simulink library "AvgModels.r2022"  (R2021b)
settings: Solver=ode45  StartTime=0.0  StopTime=10.0  RelTol=1e-3  EnableMultiTasking=on
libraries: simulink x8, $bdroot x8, slpidlib x3
(part 2 of 2)

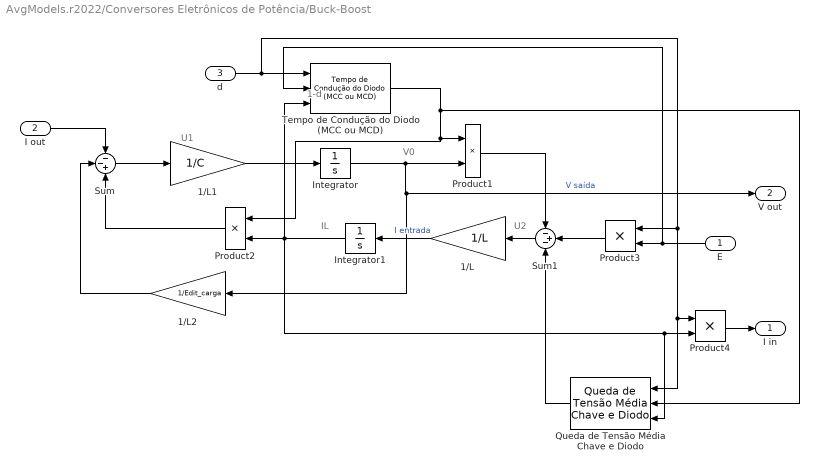
== system AvgModels.r2022/Conversores Eletrônicos de Potência/Buck-Boost ==
  note: 1-d
  note: U1
  note: V0
  note: IL
  note: U2
  E : Inport
  I out : Inport  Port=2
  d : Inport  Port=3
  1/L : Gain  Gain=1/L
  1/L1 : Gain  Gain=1/C
  1/L2 : Gain  Gain=1/Edit_carga
  Integrator : Integrator  InitialCondition=Vini  LimitOutput=on  LowerSaturationLimit=0
  Integrator1 : Integrator  InitialCondition=Iini  LimitOutput=on  LowerSaturationLimit=0
  Product{1..4} (4 alike) : Product  RndMeth=Zero
  Queda de Tensão Média Chave e Diodo : $bdroot/Conversores Eletrônicos de Potência/Queda de Tensão Média Chave e Diodo  Rswitch=Rdson  Uswitch=Vson  Rdiode=Rdon  Udiode=Vdon  direction=1
  Sum : Sum  Inputs=--+
  Sum1 : Sum  Inputs=-+-
  Tempo de Condução do Diodo (MCC ou MCD) : $bdroot/Conversores Eletrônicos de Potência/Tempo de Condução  do Diodo (MCC ou MCD)  L=L  Fs=Fs
  I in : Outport
  V out : Outport  Port=2
  wires:
  I out/1 -> Sum/1
  Sum/1 -> 1/L1/1
  Integrator/1 -> 1/L2/1, V out/1, Product1/2  "V saída"
  Product1/1 -> Sum1/1
  Sum1/1 -> 1/L/1
  1/L/1 -> Integrator1/1  "I entrada"
  Product2/1 -> Sum/3
  1/L1/1 -> Integrator/1
  Integrator1/1 -> Tempo de Condução do Diodo (MCC ou MCD)/3, Queda de Tensão Média Chave e Diodo/3, Product4/2, Product2/2
  Product3/1 -> Sum1/2
  d/1 -> Tempo de Condução do Diodo (MCC ou MCD)/1, Queda de Tensão Média Chave e Diodo/1, Product4/1, Product3/1
  Tempo de Condução do Diodo (MCC ou MCD)/1 -> Queda de Tensão Média Chave e Diodo/2, Product2/1, Product1/1
  Product4/1 -> I in/1
  E/1 -> Tempo de Condução do Diodo (MCC ou MCD)/2, Product3/2
  Queda de Tensão Média Chave e Diodo/1 -> Sum1/3
  1/L2/1 -> Sum/2

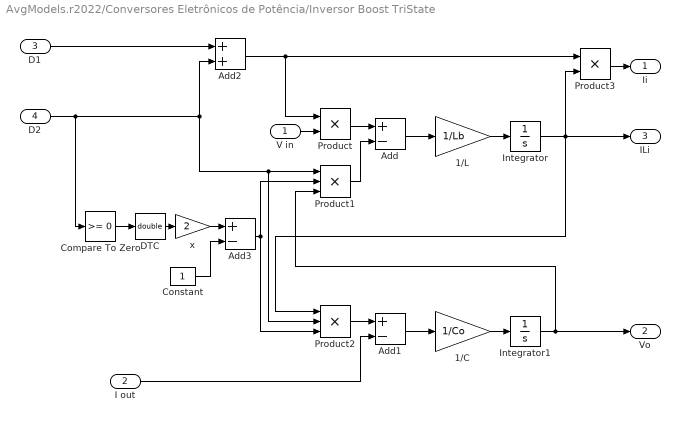
== system AvgModels.r2022/Conversores Eletrônicos de Potência/Inversor Boost TriState ==
  V in : Inport
  I out : Inport  Port=2
  D1 : Inport  Port=3
  D2 : Inport  Port=4
  1/C : Gain  Gain=1/Co
  1/L : Gain  Gain=1/Lb
  Add : Sum  Inputs=+-
  Add1 : Sum  Inputs=+-
  Add2 : Sum  Inputs=2
  Add3 : Sum  Inputs=+-
  Compare To Zero : simulink/Logic and Bit Operations/Compare To Zero  relop=>=  OutDataTypeStr=boolean
  Constant : Constant
  DTC : DataTypeConversion  OutDataTypeStr=double
  Integrator : Integrator  InitialCondition=ILb  LimitOutput=on  LowerSaturationLimit=0
  Integrator1 : Integrator  InitialCondition=Vco  LowerSaturationLimit=0
  Product : Product  RndMeth=Zero
  Product1 : Product  Inputs=3  RndMeth=Zero
  Product2 : Product  Inputs=3  RndMeth=Zero
  Product3 : Product  RndMeth=Zero
  x : Gain  Gain=2  OutDataTypeStr=double  RndMeth=Round
  Ii : Outport
  Vo : Outport  Port=2
  ILi : Outport  Port=3
  wires:
  D1/1 -> Add2/1
  V in/1 -> Product/2
  Compare To Zero/1 -> DTC/1
  Product/1 -> Add/1
  Product1/1 -> Add/2
  Add/1 -> 1/L/1
  1/L/1 -> Integrator/1
  Integrator/1 -> ILi/1, Product2/1, Product3/2
  Product2/1 -> Add1/1
  I out/1 -> Add1/2
  1/C/1 -> Integrator1/1
  Add1/1 -> 1/C/1
  Integrator1/1 -> Vo/1, Product1/3
  Product3/1 -> Ii/1
  Add2/1 -> Product/1, Product3/1
  x/1 -> Add3/1
  Add3/1 -> Product1/2, Product2/3
  Constant/1 -> Add3/2
  DTC/1 -> x/1
  D2/1 -> Compare To Zero/1, Product2/2, Product1/1, Add2/2

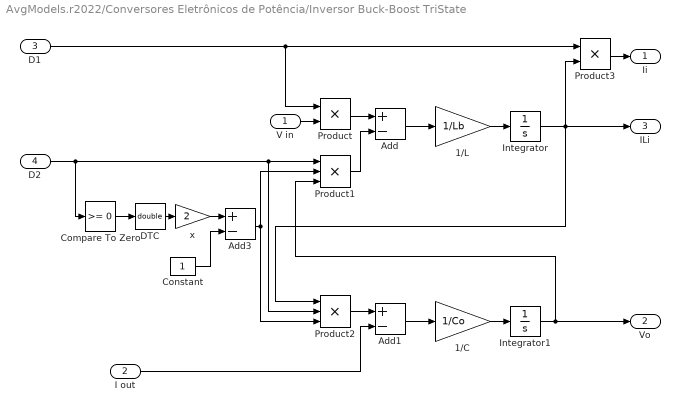
== system AvgModels.r2022/Conversores Eletrônicos de Potência/Inversor Buck-Boost TriState ==
  V in : Inport
  I out : Inport  Port=2
  D1 : Inport  Port=3
  D2 : Inport  Port=4
  1/C : Gain  Gain=1/Co
  1/L : Gain  Gain=1/Lb
  Add : Sum  Inputs=+-
  Add1 : Sum  Inputs=+-
  Add3 : Sum  Inputs=+-
  Compare To Zero : simulink/Logic and Bit Operations/Compare To Zero  relop=>=  OutDataTypeStr=boolean
  Constant : Constant
  DTC : DataTypeConversion  OutDataTypeStr=double
  Integrator : Integrator  InitialCondition=ILb  LimitOutput=on  LowerSaturationLimit=0
  Integrator1 : Integrator  InitialCondition=Vco  LowerSaturationLimit=0
  Product : Product  RndMeth=Zero
  Product1 : Product  Inputs=3  RndMeth=Zero
  Product2 : Product  Inputs=3  RndMeth=Zero
  Product3 : Product  RndMeth=Zero
  x : Gain  Gain=2  OutDataTypeStr=double  RndMeth=Round
  Ii : Outport
  Vo : Outport  Port=2
  ILi : Outport  Port=3
  wires:
  D2/1 -> Product1/1, Product2/2, Compare To Zero/1
  DTC/1 -> x/1
  Constant/1 -> Add3/2
  Add3/1 -> Product2/3, Product1/2
  x/1 -> Add3/1
  D1/1 -> Product3/1, Product/1
  Product3/1 -> Ii/1
  Integrator1/1 -> Product1/3, Vo/1
  Add1/1 -> 1/C/1
  1/C/1 -> Integrator1/1
  I out/1 -> Add1/2
  Product2/1 -> Add1/1
  Integrator/1 -> Product3/2, Product2/1, ILi/1
  1/L/1 -> Integrator/1
  Add/1 -> 1/L/1
  Product1/1 -> Add/2
  Product/1 -> Add/1
  Compare To Zero/1 -> DTC/1
  V in/1 -> Product/2

== system AvgModels.r2022/Conversores Eletrônicos de Potência/Inversor VSI ==
  V in : Inport
  I out : Inport  Port=2
  m : Inport  Port=3
  1/C : Gain  Gain=1/Co
  1/L : Gain  Gain=1/Lb
  Add : Sum  Inputs=+--
  Add1 : Sum  Inputs=+-
  Integrator : Integrator  InitialCondition=ILb  LowerSaturationLimit=0
  Integrator1 : Integrator  InitialCondition=Vco  LowerSaturationLimit=0
  Product : Product  RndMeth=Zero
  Product3 : Product  RndMeth=Zero
  Rl : Gain  Gain=Rl
  Ii : Outport
  Vo : Outport  Port=2
  ILi : Outport  Port=3
  wires:
  m/1 -> Product3/1, Product/1
  Product3/1 -> Ii/1
  Add1/1 -> 1/C/1
  1/C/1 -> Integrator1/1
  I out/1 -> Add1/2
  Integrator/1 -> Rl/1, Add1/1, Product3/2, ILi/1
  1/L/1 -> Integrator/1
  Add/1 -> 1/L/1
  Integrator1/1 -> Add/2, Vo/1
  Product/1 -> Add/1
  V in/1 -> Product/2
  Rl/1 -> Add/3

== system AvgModels.r2022/Conversores Eletrônicos de Potência/Queda de Tensão Média Chave e Diodo ==
  D1 : Inport
  D2 : Inport  Port=2
  IL : Inport  Port=3
  Bias : Bias  Bias=Uswitch
  Bias1 : Bias  Bias=Udiode
  Constant1 : Constant  Value=direction
  Product1 : Product  Inputs=3  RndMeth=Zero
  Product3 : Product  Inputs=3  RndMeth=Zero
  Sum3 : Sum  Inputs=|++
  rd : Gain  Gain=Rdiode
  rs : Gain  Gain=Rswitch
  Queda : Outport
  wires:
  Constant1/1 -> Product1/1, Product3/1
  D1/1 -> Product3/2
  IL/1 -> rd/1, rs/1
  rs/1 -> Bias/1
  rd/1 -> Bias1/1
  Bias/1 -> Product3/3
  D2/1 -> Product1/2
  Bias1/1 -> Product1/3
  Product3/1 -> Sum3/1
  Product1/1 -> Sum3/2
  Sum3/1 -> Queda/1  "D2"

== system AvgModels.r2022/Conversores Eletrônicos de Potência/Tempo de Condução do Diodo (MCC ou MCD) ==
  D1 : Inport
  Uup : Inport  Port=2
  IL : Inport  Port=3
  0 a 1 : Saturate  UpperLimit=1  LowerLimit=0
  L/Ts : Gain  Gain=2*(L*Fs)
  Product4 : Product  Inputs=/*/  RndMeth=Zero
  Saturation : Saturate  UpperLimit=1  LowerLimit=eps
  Saturation1 : Saturate  UpperLimit=inf  LowerLimit=eps
  Sum3 : Sum  Inputs=-+|
  D2 : Outport
  wires:
  IL/1 -> L/Ts/1
  L/Ts/1 -> Product4/2
  Uup/1 -> Saturation1/1
  D1/1 -> Sum3/1, Saturation/1
  Product4/1 -> 0 a 1/1  "D2+D1"
  Saturation1/1 -> Product4/1
  Saturation/1 -> Product4/3
  0 a 1/1 -> Sum3/2
  Sum3/1 -> D2/1  "D2"

== system AvgModels.r2022/MPPT/MPPT Climbing Hill ==
  V : Inport
  I : Inport  Port=2
  -Passo : Constant  Value=-1*Passo
  Int : Integrator  InitialCondition=Inicial  LimitOutput=on  UpperSaturationLimit=limsup  LowerSaturationLimit=liminf
  Sinal : Signum  ZeroCross=off
  dP/dt : TransferFcn  Numerator=[1 0]  Denominator=[1/fb 1]
  dV/dt : TransferFcn  Numerator=[1 0]  Denominator=[1/fb 1]
  x : Product  RndMeth=Zero
  x2 : Product  RndMeth=Zero
  x3 : Product  RndMeth=Zero
  Comando : Outport
  wires:
  x/1 -> dP/dt/1
  dP/dt/1 -> x2/1
  dV/dt/1 -> x2/2
  V/1 -> dV/dt/1, x/2
  I/1 -> x/1
  x2/1 -> Sinal/1
  -Passo/1 -> x3/1
  Sinal/1 -> x3/2
  x3/1 -> Int/1
  Int/1 -> Comando/1

== system AvgModels.r2022/MPPT/MPPT InC ==
  V : Inport
  I : Inport  Port=2
  -Passo : Constant  Value=-1*Passo
  Abs : Abs
  Int : Integrator  LimitOutput=on  UpperSaturationLimit=limsup  LowerSaturationLimit=liminf
  Product : Product
  Saturation : Saturate  UpperLimit=1e3  LowerLimit=0.01
  Saturation1 : Saturate  UpperLimit=1e3  LowerLimit=1e-5
  Sign : Signum
  Sinal : Signum
  Soma : Sum  Inputs=2
  dI/dt : TransferFcn  Numerator=[1 0]  Denominator=[1/fb 1]
  dV/dt : TransferFcn  Numerator=[1 0]  Denominator=[1/fb 1]
  x1 : Product  Inputs=*/  RndMeth=Zero
  x3 : Product  RndMeth=Zero
  x4 : Product  Inputs=*/  RndMeth=Zero
  Comando : Outport
  wires:
  Int/1 -> Comando/1
  x3/1 -> Int/1
  Sinal/1 -> x3/2
  -Passo/1 -> x3/1
  V/1 -> dV/dt/1, Saturation/1
  I/1 -> dI/dt/1, x4/1
  dI/dt/1 -> x1/1
  x4/1 -> Soma/1
  Saturation/1 -> x4/2
  Soma/1 -> Sinal/1
  x1/1 -> Soma/2
  Product/1 -> x1/2
  dV/dt/1 -> Sign/1, Abs/1
  Abs/1 -> Saturation1/1
  Saturation1/1 -> Product/1
  Sign/1 -> Product/2

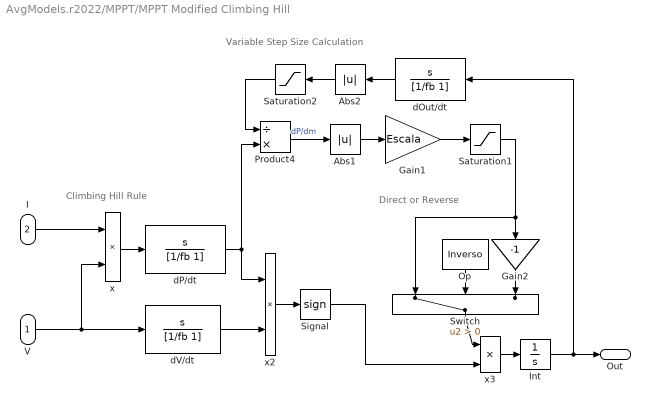
== system AvgModels.r2022/MPPT/MPPT Modified Climbing Hill ==
  note: Variable Step Size Calculation
  note: Direct or Reverse
  note: Climbing Hill Rule
  V : Inport
  I : Inport  Port=2
  Abs1 : Abs
  Abs2 : Abs
  Gain1 : Gain  Gain=Escala
  Gain2 : Gain  Gain=-1
  Int : Integrator  InitialCondition=Inicial  LimitOutput=on  UpperSaturationLimit=limsup  LowerSaturationLimit=liminf
  Op : Constant  Value=Inverso
  Product4 : Product  Inputs=/*  RndMeth=Zero
  Saturation1 : Saturate  UpperLimit=Passomax  LowerLimit=Passomin
  Saturation2 : Saturate  UpperLimit=10000  LowerLimit=0.1
  Signal : Signum
  Switch : Switch  Criteria=u2 > Threshold
  dOut/dt : TransferFcn  Numerator=[1 0]  Denominator=[1/fb 1]
  dP/dt : TransferFcn  Numerator=[1 0]  Denominator=[1/fb 1]
  dV/dt : TransferFcn  Numerator=[1 0]  Denominator=[1/fb 1]
  x : Product  RndMeth=Zero
  x2 : Product  RndMeth=Zero
  x3 : Product  RndMeth=Zero
  Out : Outport
  wires:
  Int/1 -> Out/1, dOut/dt/1
  x3/1 -> Int/1
  Signal/1 -> x3/2
  x2/1 -> Signal/1
  I/1 -> x/1
  V/1 -> dV/dt/1, x/2
  dV/dt/1 -> x2/2
  dP/dt/1 -> x2/1, Product4/2
  x/1 -> dP/dt/1
  Saturation1/1 -> Gain2/1, Switch/1
  Abs1/1 -> Gain1/1
  dOut/dt/1 -> Abs2/1
  Product4/1 -> Abs1/1  "dP/dm"
  Gain1/1 -> Saturation1/1
  Abs2/1 -> Saturation2/1
  Saturation2/1 -> Product4/1
  Switch/1 -> x3/1
  Op/1 -> Switch/2
  Gain2/1 -> Switch/3

== system AvgModels.r2022/MPPT/MPPT Oscillation ==
  V : Inport
  Abs : Abs
  Add : Sum  Inputs=+-
  K0 : Gain  Gain=K0
  PID Controller : slpidlib/PID Controller  Controller=PID  Form=Parallel  TimeDomain=Continuous-time  UseExternalTs=off  SampleTime=-1  IntegratorMethod=Forward Euler  FilterMethod=Forward Euler  ControllerParametersSource=internal  P=Kp  I=Ki  D=0  UseFilter=on  N=100  TunerSelectOption=Transfer Function Based (PID Tuner App)  InitialConditionSource=internal  InitialConditionForIntegrator=0  InitialConditionForFilter=0  DifferentiatorICPrevScaledInput=0  ExternalReset=none  TrackingMode=off  Kt=1  LimitOutput=on  SatLimitsSource=internal  UpperSaturationLimit=limsup  LowerSaturationLimit=liminf  LinearizeAsGain=on  AntiWindupMode=clamping  Kb=1  POutMin=[]  POutMax=[]  IOutMin=[]  IOutMax=[]  DOutMin=[]  DOutMax=[]  NOutMin=[]  NOutMax=[]  SumOutMin=[]  SumOutMax=[]  SaturationOutMin=[]  SaturationOutMax=[]  PParamMin=[]  PParamMax=[]  IParamMin=[]  IParamMax=[]  DParamMin=[]  DParamMax=[]  NParamMin=[]  NParamMax=[]  KbParamMin=[]  KbParamMax=[]  KtParamMin=[]  KtParamMax=[]  KbOutMin=[]  KbOutMax=[]  KtOutMin=[]  KtOutMax=[]  IntegratorOutMin=[]  IntegratorOutMax=[]  FilterOutMin=[]  FilterOutMax=[]  SumI1OutMin=[]  SumI1OutMax=[]  SumI2OutMin=[]  SumI2OutMax=[]  SumI3OutMin=[]  SumI3OutMax=[]  SumI4OutMin=[]  SumI4OutMax=[]  SumDOutMin=[]  SumDOutMax=[]  DifferentiatorOutMin=[]  DifferentiatorOutMax=[]  FilterDiffOutCoefMin=[]  FilterDiffOutCoefMax=[]  ReciprocalOutMin=[]  ReciprocalOutMax=[]  SumDenOutMin=[]  SumDenOutMax=[]  SumNumOutMin=[]  SumNumOutMax=[]  DivideOutMin=[]  DivideOutMax=[]  UdiffTsProdOutMin=[]  UdiffTsProdOutMax=[]  NTsProdOutMin=[]  NTsProdOutMax=[]  UintegralTsProdOutMin=[]  UintegralTsProdOutMax=[]  UngainTsProdOutMin=[]  UngainTsProdOutMax=[]  IntegratorContinuousStateAttributes=''  IntegratorStateMustResolveToSignalObject=off  IntegratorRTWStateStorageClass=Auto  FilterContinuousStateAttributes=''  FilterStateMustResolveToSignalObject=off  FilterRTWStateStorageClass=Auto  ParallelPVariant=InternalParameters  IdealPVariant=Disabled  IVariant=InternalParameters  DVariant=InternalParameters  IntegratorVariant=Continuous  SatVariant=Enabled  AWVariant=ContClampingParallel  PCopyVariant=Disabled  TRVariant=Disabled  FdbkBlocksVariant=Forward  IdealPFdbkVariant=Disabled  SatFdbkVariant=Disabled  DerivativeFilterVariant=ContFilter  NVariant=InternalParameters  NCopyVariant=Disabled  FilterICVariant=InternalICsFilter  IntegratorICVariant=InternalICs  ExternalResetVariant=Disabled  TRSumVariant=Passthrough  SumFdbkVariant=Disabled  SumVariant=Sum_PID  TsampFilterVariant=InternalTs  TsampNgainVariant=Passthrough  TsampIntegralVariant=Passthrough  ExternalSaturationOutDataTypeStr=Inherit: Same as second input
  Passa Baixa : TransferFcn  Numerator=[wbaixa]  Denominator=[1 wbaixa]
  Passa Baixa2 : TransferFcn  Numerator=[wbaixa]  Denominator=[1 wbaixa]
  Passa Banda : ZeroPole  Zeros=[0]  Poles=[-wbaixa -walta]  Gain=[wbaixa]
  Comando : Outport
  wires:
  Add/1 -> PID Controller/1
  PID Controller/1 -> Comando/1
  Passa Baixa/1 -> K0/1
  Passa Banda/1 -> Abs/1
  Abs/1 -> Passa Baixa2/1
  Passa Baixa2/1 -> Add/2
  V/1 -> Passa Banda/1, Passa Baixa/1
  K0/1 -> Add/1

== system AvgModels.r2022/MPPT/MPPT V constante ==
  V : Inport
  PID Controller : slpidlib/PID Controller  Controller=PID  Form=Parallel  TimeDomain=Continuous-time  UseExternalTs=off  SampleTime=-1  IntegratorMethod=Forward Euler  FilterMethod=Forward Euler  ControllerParametersSource=internal  P=Kp  I=Ki  D=0  UseFilter=on  N=100  TunerSelectOption=Transfer Function Based (PID Tuner App)  InitialConditionSource=internal  InitialConditionForIntegrator=0  InitialConditionForFilter=0  DifferentiatorICPrevScaledInput=0  ExternalReset=none  TrackingMode=off  Kt=1  LimitOutput=on  SatLimitsSource=internal  UpperSaturationLimit=limsup  LowerSaturationLimit=liminf  LinearizeAsGain=on  AntiWindupMode=clamping  Kb=1  POutMin=[]  POutMax=[]  IOutMin=[]  IOutMax=[]  DOutMin=[]  DOutMax=[]  NOutMin=[]  NOutMax=[]  SumOutMin=[]  SumOutMax=[]  SaturationOutMin=[]  SaturationOutMax=[]  PParamMin=[]  PParamMax=[]  IParamMin=[]  IParamMax=[]  DParamMin=[]  DParamMax=[]  NParamMin=[]  NParamMax=[]  KbParamMin=[]  KbParamMax=[]  KtParamMin=[]  KtParamMax=[]  KbOutMin=[]  KbOutMax=[]  KtOutMin=[]  KtOutMax=[]  IntegratorOutMin=[]  IntegratorOutMax=[]  FilterOutMin=[]  FilterOutMax=[]  SumI1OutMin=[]  SumI1OutMax=[]  SumI2OutMin=[]  SumI2OutMax=[]  SumI3OutMin=[]  SumI3OutMax=[]  SumI4OutMin=[]  SumI4OutMax=[]  SumDOutMin=[]  SumDOutMax=[]  DifferentiatorOutMin=[]  DifferentiatorOutMax=[]  FilterDiffOutCoefMin=[]  FilterDiffOutCoefMax=[]  ReciprocalOutMin=[]  ReciprocalOutMax=[]  SumDenOutMin=[]  SumDenOutMax=[]  SumNumOutMin=[]  SumNumOutMax=[]  DivideOutMin=[]  DivideOutMax=[]  UdiffTsProdOutMin=[]  UdiffTsProdOutMax=[]  NTsProdOutMin=[]  NTsProdOutMax=[]  UintegralTsProdOutMin=[]  UintegralTsProdOutMax=[]  UngainTsProdOutMin=[]  UngainTsProdOutMax=[]  IntegratorContinuousStateAttributes=''  IntegratorStateMustResolveToSignalObject=off  IntegratorRTWStateStorageClass=Auto  FilterContinuousStateAttributes=''  FilterStateMustResolveToSignalObject=off  FilterRTWStateStorageClass=Auto  ParallelPVariant=InternalParameters  IdealPVariant=Disabled  IVariant=InternalParameters  DVariant=InternalParameters  IntegratorVariant=Continuous  SatVariant=Enabled  AWVariant=ContClampingParallel  PCopyVariant=Disabled  TRVariant=Disabled  FdbkBlocksVariant=Forward  IdealPFdbkVariant=Disabled  SatFdbkVariant=Disabled  DerivativeFilterVariant=ContFilter  NVariant=InternalParameters  NCopyVariant=Disabled  FilterICVariant=InternalICsFilter  IntegratorICVariant=InternalICs  ExternalResetVariant=Disabled  TRSumVariant=Passthrough  SumFdbkVariant=Disabled  SumVariant=Sum_PID  TsampFilterVariant=InternalTs  TsampNgainVariant=Passthrough  TsampIntegralVariant=Passthrough  ExternalSaturationOutDataTypeStr=Inherit: Same as second input
  Sub : Sum  Inputs=+-
  Vref = 0.78.Voc : Constant  Value=Voc*0.78
  Comando : Outport
  wires:
  PID Controller/1 -> Comando/1
  V/1 -> Sub/1
  Sub/1 -> PID Controller/1
  Vref = 0.78.Voc/1 -> Sub/2

== system AvgModels.r2022/MPPT/MPPT beta ==
  V : Inport
  I : Inport  Port=2
  Abs : Abs
  Add : Sum  Inputs=|+-
  Add1 : Sum  Inputs=+-
  Beta ref : Constant  Value=betaref
  Divide : Product  Inputs=*/
  PID Controller : slpidlib/PID Controller  Controller=PID  Form=Parallel  TimeDomain=Continuous-time  UseExternalTs=off  SampleTime=-1  IntegratorMethod=Forward Euler  FilterMethod=Forward Euler  ControllerParametersSource=internal  P=Kp  I=Ki  D=0  UseFilter=on  N=100  TunerSelectOption=Transfer Function Based (PID Tuner App)  InitialConditionSource=internal  InitialConditionForIntegrator=0  InitialConditionForFilter=0  DifferentiatorICPrevScaledInput=0  ExternalReset=none  TrackingMode=off  Kt=1  LimitOutput=on  SatLimitsSource=internal  UpperSaturationLimit=limsup  LowerSaturationLimit=liminf  LinearizeAsGain=on  AntiWindupMode=clamping  Kb=1  POutMin=[]  POutMax=[]  IOutMin=[]  IOutMax=[]  DOutMin=[]  DOutMax=[]  NOutMin=[]  NOutMax=[]  SumOutMin=[]  SumOutMax=[]  SaturationOutMin=[]  SaturationOutMax=[]  PParamMin=[]  PParamMax=[]  IParamMin=[]  IParamMax=[]  DParamMin=[]  DParamMax=[]  NParamMin=[]  NParamMax=[]  KbParamMin=[]  KbParamMax=[]  KtParamMin=[]  KtParamMax=[]  KbOutMin=[]  KbOutMax=[]  KtOutMin=[]  KtOutMax=[]  IntegratorOutMin=[]  IntegratorOutMax=[]  FilterOutMin=[]  FilterOutMax=[]  SumI1OutMin=[]  SumI1OutMax=[]  SumI2OutMin=[]  SumI2OutMax=[]  SumI3OutMin=[]  SumI3OutMax=[]  SumI4OutMin=[]  SumI4OutMax=[]  SumDOutMin=[]  SumDOutMax=[]  DifferentiatorOutMin=[]  DifferentiatorOutMax=[]  FilterDiffOutCoefMin=[]  FilterDiffOutCoefMax=[]  ReciprocalOutMin=[]  ReciprocalOutMax=[]  SumDenOutMin=[]  SumDenOutMax=[]  SumNumOutMin=[]  SumNumOutMax=[]  DivideOutMin=[]  DivideOutMax=[]  UdiffTsProdOutMin=[]  UdiffTsProdOutMax=[]  NTsProdOutMin=[]  NTsProdOutMax=[]  UintegralTsProdOutMin=[]  UintegralTsProdOutMax=[]  UngainTsProdOutMin=[]  UngainTsProdOutMax=[]  IntegratorContinuousStateAttributes=''  IntegratorStateMustResolveToSignalObject=off  IntegratorRTWStateStorageClass=Auto  FilterContinuousStateAttributes=''  FilterStateMustResolveToSignalObject=off  FilterRTWStateStorageClass=Auto  ParallelPVariant=InternalParameters  IdealPVariant=Disabled  IVariant=InternalParameters  DVariant=InternalParameters  IntegratorVariant=Continuous  SatVariant=Enabled  AWVariant=ContClampingParallel  PCopyVariant=Disabled  TRVariant=Disabled  FdbkBlocksVariant=Forward  IdealPFdbkVariant=Disabled  SatFdbkVariant=Disabled  DerivativeFilterVariant=ContFilter  NVariant=InternalParameters  NCopyVariant=Disabled  FilterICVariant=InternalICsFilter  IntegratorICVariant=InternalICs  ExternalResetVariant=Disabled  TRSumVariant=Passthrough  SumFdbkVariant=Disabled  SumVariant=Sum_PID  TsampFilterVariant=InternalTs  TsampNgainVariant=Passthrough  TsampIntegralVariant=Passthrough  ExternalSaturationOutDataTypeStr=Inherit: Same as second input
  c : Gain  Gain=1.60217646e-19/(1*1.3806503e-23*303.15*54)
  ln : Math  Operator=log  SignedPower=on  SaturateOnIntegerOverflow=on
  sat : Saturate  UpperLimit=inf  LowerLimit=1
  sat1 : Saturate  UpperLimit=inf  LowerLimit=0.1
  Comando : Outport
  wires:
  Add/1 -> PID Controller/1
  PID Controller/1 -> Comando/1
  Beta ref/1 -> Add/1
  I/1 -> Abs/1
  Divide/1 -> ln/1
  V/1 -> c/1, sat/1
  c/1 -> Add1/2
  Add1/1 -> Add/2  "Beta"
  sat/1 -> Divide/2
  ln/1 -> Add1/1
  Abs/1 -> sat1/1
  sat1/1 -> Divide/1

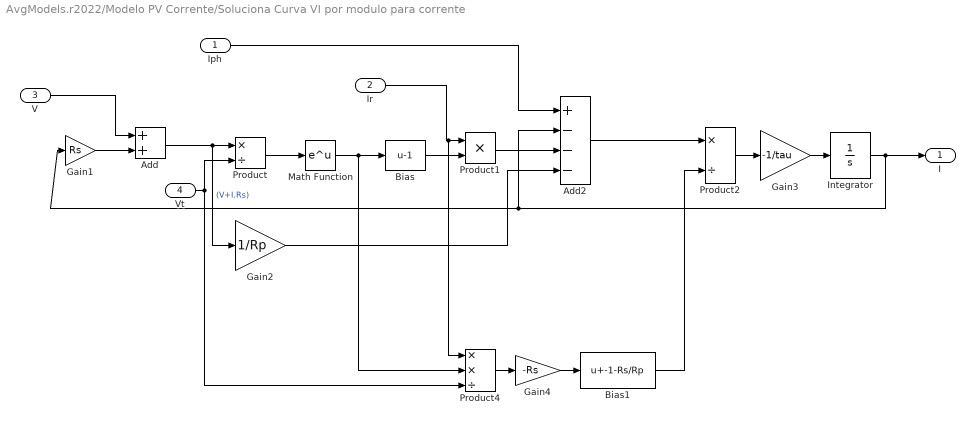
== system AvgModels.r2022/Modelo PV Corrente/Soluciona Curva VI por modulo para corrente ==
  Iph : Inport
  Ir : Inport  Port=2
  V : Inport  Port=3
  Vt : Inport  Port=4
  Add : Sum
  Add2 : Sum  Inputs=+---
  Bias : Bias  Bias=-1
  Bias1 : Bias  Bias=-1-Rs/Rp
  Gain1 : Gain  Gain=Rs
  Gain2 : Gain  Gain=1/Rp
  Gain3 : Gain  Gain=-1/tau
  Gain4 : Gain  Gain=-Rs
  Integrator : Integrator  LimitOutput=on  LowerSaturationLimit=0
  Math Function : Math  SignedPower=on  SaturateOnIntegerOverflow=on
  Product : Product  Inputs=*/
  Product1 : Product
  Product2 : Product  Inputs=*/
  Product4 : Product  Inputs=**/
  I : Outport
  wires:
  Integrator/1 -> I/1, Add2/2, Gain1/1
  Add2/1 -> Product2/1
  Product1/1 -> Add2/3
  Iph/1 -> Add2/1
  Bias/1 -> Product1/2
  Product/1 -> Math Function/1
  Add/1 -> Product/1, Gain2/1  "(V+I.Rs)"
  Gain1/1 -> Add/2
  Product2/1 -> Gain3/1
  Gain2/1 -> Add2/4
  Gain3/1 -> Integrator/1
  Vt/1 -> Product/2, Product4/3
  Math Function/1 -> Product4/2, Bias/1
  Ir/1 -> Product4/1, Product1/1
  Product4/1 -> Gain4/1
  Gain4/1 -> Bias1/1
  Bias1/1 -> Product2/2
  V/1 -> Add/1

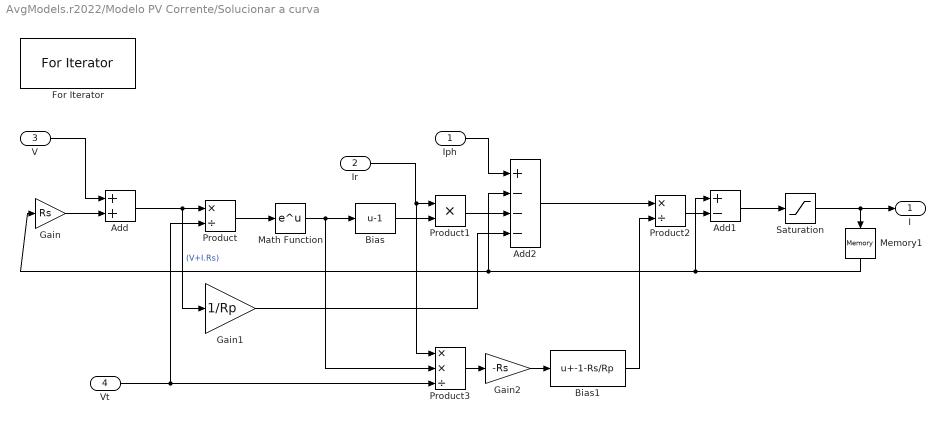
== system AvgModels.r2022/Modelo PV Corrente/Solucionar a curva ==
  Iph : Inport
  Ir : Inport  Port=2
  V : Inport  Port=3
  Vt : Inport  Port=4
  Add : Sum
  Add1 : Sum  Inputs=+-
  Add2 : Sum  Inputs=+---
  Bias : Bias  Bias=-1
  Bias1 : Bias  Bias=-1-Rs/Rp
  For Iterator : ForIterator  IterationLimit=3  ShowIterationPort=off
  Gain : Gain  Gain=Rs
  Gain1 : Gain  Gain=1/Rp
  Gain2 : Gain  Gain=-Rs
  Math Function : Math  SignedPower=on  SaturateOnIntegerOverflow=on
  Memory1 : Memory  InheritSampleTime=on
  Product : Product  Inputs=*/
  Product1 : Product
  Product2 : Product  Inputs=*/
  Product3 : Product  Inputs=**/
  Saturation : Saturate  UpperLimit=inf  LowerLimit=0
  I : Outport
  wires:
  Add1/1 -> Saturation/1
  Gain/1 -> Add/2
  V/1 -> Add/1
  Vt/1 -> Product3/3, Product/2
  Add/1 -> Gain1/1, Product/1  "(V+I.Rs)"
  Product/1 -> Math Function/1
  Math Function/1 -> Product3/2, Bias/1
  Bias/1 -> Product1/2
  Ir/1 -> Product3/1, Product1/1
  Iph/1 -> Add2/1
  Product1/1 -> Add2/3
  Gain1/1 -> Add2/4
  Add2/1 -> Product2/1
  Product2/1 -> Add1/2
  Product3/1 -> Gain2/1
  Gain2/1 -> Bias1/1
  Bias1/1 -> Product2/2
  Saturation/1 -> Memory1/1, I/1
  Memory1/1 -> Add1/1, Gain/1, Add2/2

== system AvgModels.r2022/Modelo PV Tensão/Soluciona Curva VI por modulo ==
  Ir : Inport
  Iph : Inport  Port=2
  Ipv : Inport  Port=3
  Vt : Inport  Port=4
  Add : Sum
  Add1 : Sum  Inputs=--
  Add2 : Sum  Inputs=+---
  Bias : Bias  Bias=-1
  Gain1 : Gain  Gain=Rs
  Gain2 : Gain  Gain=1/Rp
  Gain3 : Gain  Gain=-1/tau
  Integrator : Integrator  LimitOutput=on  LowerSaturationLimit=0
  Math Function : Math  SignedPower=on  SaturateOnIntegerOverflow=on
  Product : Product  Inputs=*/
  Product1 : Product
  Product2 : Product  Inputs=*/
  Product3 : Product  Inputs=**/
  Vpv : Outport
  wires:
  Ipv/1 -> Gain1/1, Add2/2
  Add2/1 -> Product2/1
  Product1/1 -> Add2/3
  Iph/1 -> Add2/1
  Ir/1 -> Product3/1, Product1/1
  Bias/1 -> Product1/2
  Math Function/1 -> Product3/2, Bias/1
  Product/1 -> Math Function/1
  Add/1 -> Product/1, Gain2/1  "(V+I.Rs)"
  Vt/1 -> Product3/3, Product/2
  Integrator/1 -> Vpv/1, Add/1
  Gain1/1 -> Add/2
  Product2/1 -> Gain3/1
  Product3/1 -> Add1/1
  Gain2/1 -> Add2/4, Add1/2
  Add1/1 -> Product2/2
  Gain3/1 -> Integrator/1

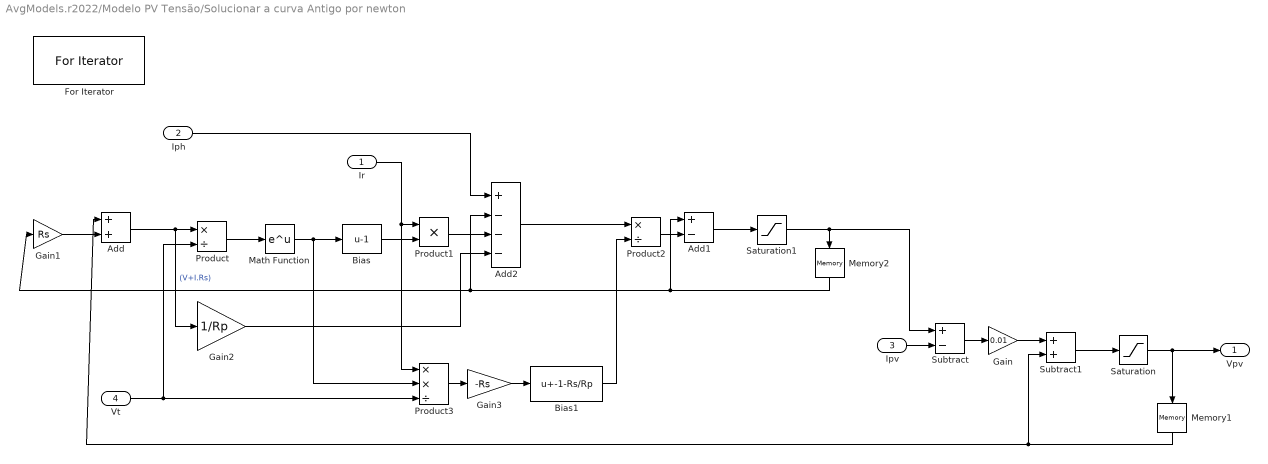
== system AvgModels.r2022/Modelo PV Tensão/Solucionar a curva Antigo por newton ==
  Ir : Inport
  Iph : Inport  Port=2
  Ipv : Inport  Port=3
  Vt : Inport  Port=4
  Add : Sum
  Add1 : Sum  Inputs=+-
  Add2 : Sum  Inputs=+---
  Bias : Bias  Bias=-1
  Bias1 : Bias  Bias=-1-Rs/Rp
  For Iterator : ForIterator  IterationLimit=4  ShowIterationPort=off
  Gain : Gain  Gain=0.01
  Gain1 : Gain  Gain=Rs
  Gain2 : Gain  Gain=1/Rp
  Gain3 : Gain  Gain=-Rs
  Math Function : Math  SignedPower=on  SaturateOnIntegerOverflow=on
  Memory1 : Memory  InitialCondition=Voc  InheritSampleTime=on
  Memory2 : Memory  InheritSampleTime=on
  Product : Product  Inputs=*/
  Product1 : Product
  Product2 : Product  Inputs=*/
  Product3 : Product  Inputs=**/
  Saturation : Saturate  UpperLimit=inf  LowerLimit=0
  Saturation1 : Saturate  UpperLimit=inf  LowerLimit=0
  Subtract : Sum  Inputs=+-
  Subtract1 : Sum
  Vpv : Outport
  wires:
  Subtract1/1 -> Saturation/1
  Ipv/1 -> Subtract/2
  Subtract/1 -> Gain/1
  Gain/1 -> Subtract1/1
  Saturation/1 -> Vpv/1, Memory1/1
  Memory2/1 -> Add2/2, Gain1/1, Add1/1
  Saturation1/1 -> Subtract/1, Memory2/1
  Bias1/1 -> Product2/2
  Gain3/1 -> Bias1/1
  Product3/1 -> Gain3/1
  Product2/1 -> Add1/2
  Add2/1 -> Product2/1
  Gain2/1 -> Add2/4
  Product1/1 -> Add2/3
  Iph/1 -> Add2/1
  Ir/1 -> Product3/1, Product1/1
  Bias/1 -> Product1/2
  Math Function/1 -> Bias/1, Product3/2
  Product/1 -> Math Function/1
  Add/1 -> Product/1, Gain2/1  "(V+I.Rs)"
  Vt/1 -> Product/2, Product3/3
  Memory1/1 -> Add/1, Subtract1/2
  Gain1/1 -> Add/2
  Add1/1 -> Saturation1/1

== system AvgModels.r2022/Modelo PV Tensão/Subsystem ==
  In1 : Inport
  Enable : EnablePort
  S-Function : S-Function  FunctionName=animarcurvaPV  Parameters=[Voc Isc Rp Rs Ns a]  SFunctionDeploymentMode=off  EnableBusSupport=off
  Terminator : Terminator
  wires:
  In1/1 -> S-Function/1
  S-Function/1 -> Terminator/1

== system AvgModels.r2022/Modelos Animados/Modelo Antena 1 DOF ==
  Torque : Inport
  Referência : Inport  Port=2
  Braço-Robô : TransferFcn  Numerator=[K]  Denominator=[J 1 0]
  Mux : Mux  Inputs=3
  S-Function : S-Function  FunctionName=animarantena  SFunctionDeploymentMode=off  EnableBusSupport=off
  Ângulo : Outport
  wires:
  Referência/1 -> Mux/1
  Braço-Robô/1 -> Mux/2, Ângulo/1
  Mux/1 -> S-Function/1
  Torque/1 -> Braço-Robô/1, Mux/3

== system AvgModels.r2022/Modelos Animados/Modelo Braço Robô 1 DOF ==
  Torque : Inport
  Referência : Inport  Port=2
  Braço-Robô : TransferFcn  Numerator=[K]  Denominator=[J 1 0]
  Mux : Mux  Inputs=3
  S-Function : S-Function  FunctionName=animarposicao  SFunctionDeploymentMode=off  EnableBusSupport=off
  Ângulo : Outport
  wires:
  Torque/1 -> Mux/3, Braço-Robô/1
  Mux/1 -> S-Function/1
  Braço-Robô/1 -> Ângulo/1, Mux/2
  Referência/1 -> Mux/1

== system AvgModels.r2022/Modelos Animados/Submarino Autônomo ==
  h_ref : Inport
  u : Inport  Port=2
  Animar : S-Function  FunctionName=animarUFSS  SFunctionDeploymentMode=off  EnableBusSupport=off
  Mux1 : Mux
  UFSS : Subsystem
  h : Outport
  Pitch : Outport  Port=2
  Estados : Outport  Port=3
  wires:
  h_ref/1 -> Mux1/1
  UFSS/4(x) -> Estados/1
  Mux1/1 -> Animar/1
  UFSS/2(Pitch) -> Pitch/1, Mux1/2
  u/1 -> UFSS/1(u)
  UFSS/3(Elevator) -> Mux1/3
  UFSS/1(h) -> h/1, Mux1/4

== system AvgModels.r2022/Modelos Animados/Suspensão 1 DOF ==
  x (solo) : Inport
  Atuador : Inport  Port=2
  Mux : Mux  Inputs=2
  S-Function : S-Function  FunctionName=animarsuspensao  SFunctionDeploymentMode=off  EnableBusSupport=off
  Sistema de Suspensao : Subsystem
  y (massa) : Outport
  acel : Outport  Port=2
  wires:
  Sistema de Suspensao/1(y) -> y (massa)/1, Mux/2
  x (solo)/1 -> Mux/1, Sistema de Suspensao/1(x)
  Sistema de Suspensao/2(acel) -> acel/1
  Mux/1 -> S-Function/1
  Atuador/1 -> Sistema de Suspensao/2(F)

== system AvgModels.r2022/Virtual Synchronous Machine/Modelo Elétrico ==
  Velocidade Angular do Rotor W : Inport
  Teta : Inport  Port=2
  MfIf : Inport  Port=3
  Corrente do Estator [ia,ib,ic] : Inport  Port=4
  Mux : Mux  Inputs=3
  Potencia reativa : Subsystem
  Subsystem3 : Subsystem
  Subsystem4 : Subsystem
  Tensoes Induzidas : Subsystem
  Torque eletromagnetico : Subsystem
  Te : Outport
  Q : Outport  Port=2
  Tensão Induzida [ea,eb,ec] : Outport  Port=3
  wires:
  Mux/1 -> Potencia reativa/1("[teta,teta-120,teta-240]"), Tensoes Induzidas/1("[teta,teta-120,teta-240]"), Torque eletromagnetico/1("[teta,teta-120,teta-240]")
  Subsystem4/1(teta - 240) -> Mux/3  "teta - 240"
  Subsystem3/1(teta - 120) -> Mux/2  "teta - 120"
  Corrente do Estator [ia,ib,ic]/1 -> Potencia reativa/3(Corrente do Estator [ia,ib,ic]), Torque eletromagnetico/3(Corrente do Estator [ia,ib,ic])
  Tensoes Induzidas/1(Tensão Induzida [ea,eb,ec]) -> Tensão Induzida [ea,eb,ec]/1  "Tensão Induzida [ea,eb,ec]"
  Potencia reativa/1(Q) -> Q/1  "Q"
  Torque eletromagnetico/1(Te) -> Te/1  "Te"
  Velocidade Angular do Rotor W/1 -> Tensoes Induzidas/3(Velocidade Angular do Rotor W), Potencia reativa/4(Velocidade Angular do Rotor W)  "W"
  MfIf/1 -> Potencia reativa/2(MfIf), Tensoes Induzidas/2(MfIf), Torque eletromagnetico/2(MfIf)  "Mf If"
  Teta/1 -> Subsystem4/1(teta), Subsystem3/1(teta), Mux/1  "teta"

== system AvgModels.r2022/Modelos Animados/Submarino Autônomo/UFSS ==
  u : Inport
  Atuador : TransferFcn  Numerator=[2]  Denominator=[1 2]
  Dinamica do Veículo : TransferFcn  Commented=through  Numerator=-0.125*[1 0.435]  Denominator=conv([1 1.23],[1 0.226 0.0169])
  Gain : Gain  Gain="[0   -0.1250   -0.0544]"  Multiplication=Matrix(K*u)
  Int : TransferFcn  Numerator=1  Denominator=[1 0]
  Mux : Mux
  Profundidade : TransferFcn  Numerator=0.1  Denominator=[0.1 1]
  Veículo : StateSpace  A="[-1.4560   -0.2949   -0.0208; 1.0000         0         0;    0    1.0000         0]"  B=[1 0 0]'  C=eye(3)  D=[0;0;0]  InitialCondition=0
  h : Outport
  Pitch : Outport  Port=2
  Elevator : Outport  Port=3
  x : Outport  Port=4
  wires:
  u/1 -> Atuador/1
  Atuador/1 -> Elevator/1, Veículo/1, Mux/1, Dinamica do Veículo/1
  Profundidade/1 -> Mux/3, Int/1
  Veículo/1 -> Mux/2, Gain/1
  Gain/1 -> Profundidade/1, Pitch/1
  Mux/1 -> x/1
  Int/1 -> Mux/4, h/1

== system AvgModels.r2022/Modelos Animados/Suspensão 1 DOF/Sistema de Suspensao ==
  x : Inport
  F : Inport  Port=2
  Bias : Bias  Bias=2
  Derivative1 : Derivative  CoefficientInTFapproximation=10*B
  Gain : Gain  Gain=1/M
  Gain1 : Gain  Gain=K
  Gain2 : Gain  Gain=B
  Integrator : Integrator
  Integrator1 : Integrator
  Sum1 : Sum  Inputs=+++
  Sum2 : Sum  Inputs=+|-
  y : Outport
  acel : Outport  Port=2
  wires:
  Gain1/1 -> Sum1/1  "y"
  x/1 -> Sum2/1
  Bias/1 -> y/1
  F/1 -> Sum1/3
  Integrator/1 -> Integrator1/1  "v"
  Integrator1/1 -> Bias/1, Sum2/2
  Gain/1 -> Integrator/1, acel/1  "a"
  Sum1/1 -> Gain/1  "y"
  Sum2/1 -> Gain1/1, Gain2/1
  Gain2/1 -> Derivative1/1
  Derivative1/1 -> Sum1/2

== system AvgModels.r2022/Virtual Synchronous Machine/Modelo Elétrico/Potencia reativa ==
  "[teta,teta-120,teta-240]" : Inport
  MfIf : Inport  Port=2
  Corrente do Estator [ia,ib,ic] : Inport  Port=3
  Velocidade Angular do Rotor W : Inport  Port=4
  Gain1 : Gain  Gain=-1
  Product1 : Product
  Product7 : Product  Inputs=3
  Sum3 : Sum  Inputs=+
  Trigonometric Function1 : Trigonometry  Operator=cos
  Q : Outport
  wires:
  MfIf/1 -> Product7/2
  Corrente do Estator [ia,ib,ic]/1 -> Product1/2  "ia"
  Velocidade Angular do Rotor W/1 -> Gain1/1
  "[teta,teta-120,teta-240]"/1 -> Trigonometric Function1/1  "[teta,teta-120,teta-240]"
  Product1/1 -> Sum3/1  "[ia*cos(ia*cos(teta),ib*cos(teta-120),ic*cos(teta-240)]"
  Product7/1 -> Q/1  "-W*Mf If*[ ia*cos(teta) + ib*cos(teta-120) + ic*cos(teta-240)]"
  Gain1/1 -> Product7/3  "-W"
  Trigonometric Function1/1 -> Product1/1  "cos([teta,teta-120,teta-240])"
  Sum3/1 -> Product7/1  "ia*cos(teta) + ib*cos(teta-120) + ic*cos(teta-240)"

== system AvgModels.r2022/Virtual Synchronous Machine/Modelo Elétrico/Subsystem3 ==
  teta : Inport
  -120 : Constant  Value=(2*pi)/3
  Sum : Sum  Inputs=|+-
  teta - 120 : Outport
  wires:
  Sum/1 -> teta - 120/1
  teta/1 -> Sum/1
  -120/1 -> Sum/2

== system AvgModels.r2022/Virtual Synchronous Machine/Modelo Elétrico/Subsystem4 ==
  teta : Inport
  -240 : Constant  Value=(4*pi)/3
  Sum1 : Sum  Inputs=|+-
  teta - 240 : Outport
  wires:
  teta/1 -> Sum1/1
  -240/1 -> Sum1/2
  Sum1/1 -> teta - 240/1

== system AvgModels.r2022/Virtual Synchronous Machine/Modelo Elétrico/Tensoes Induzidas ==
  "[teta,teta-120,teta-240]" : Inport
  MfIf : Inport  Port=2
  Velocidade Angular do Rotor W : Inport  Port=3
  Product8 : Product  Inputs=3
  Trigonometric Function2 : Trigonometry
  Tensão Induzida [ea,eb,ec] : Outport
  wires:
  Product8/1 -> Tensão Induzida [ea,eb,ec]/1  "[W*Mf If*sin(teta),W*Mf If*sin(teta-120),W*Mf If*sin(teta-240)]"
  MfIf/1 -> Product8/2  "Mf If"
  "[teta,teta-120,teta-240]"/1 -> Trigonometric Function2/1  "[teta,teta-120,teta-240]"
  Velocidade Angular do Rotor W/1 -> Product8/3  "W"
  Trigonometric Function2/1 -> Product8/1  "[sin(teta),sin(teta-120),sin(teta-240)]"

== system AvgModels.r2022/Virtual Synchronous Machine/Modelo Elétrico/Torque eletromagnetico ==
  "[teta,teta-120,teta-240]" : Inport
  MfIf : Inport  Port=2
  Corrente do Estator [ia,ib,ic] : Inport  Port=3
  Product : Product
  Product5 : Product
  Sum2 : Sum  Inputs=+
  Trigonometric Function : Trigonometry
  Te : Outport
  wires:
  Sum2/1 -> Product5/2  "ia*sin(teta) + ib*sin(teta-120) + ic*sin(teta-240)"
  Product5/1 -> Te/1  "Mf If * [ia*sin(teta) + ib*sin(teta-120) + ic*sin(teta-240) ]"
  Corrente do Estator [ia,ib,ic]/1 -> Product/2  "Corrente do Estator [ia,ib,ic]"
  "[teta,teta-120,teta-240]"/1 -> Trigonometric Function/1  "[teta,teta-120,teta-240]"
  Product/1 -> Sum2/1  "[ia*sin(teta),ib*sin(teta-120) ,ic*sin(teta-240)]"
  MfIf/1 -> Product5/1  "Mf If"
  Trigonometric Function/1 -> Product/1  "sin([teta,teta-120,teta-240])"
